simulink model "three_phase_full_wave_fully_controlled_rectifier_ckt_for_seperately_exiceted_dc_motor"  (R2025a)
settings: Solver=VariableStepAuto  StartTime=0.0  StopTime=.1  RelTol=1e-3
libraries: spsThyristorLib x6, spsDCVoltageSourceLib x1, spsCurrentMeasurementLib x1, spsSeriesRLCBranchLib x1, spsThreePhaseVIMeasurementLib x1, spsThreePhaseSourceLib x1, spsVoltageMeasurementLib x1, sps_lib x1
settings Model: Creator=HP  LastModifiedBy=samar

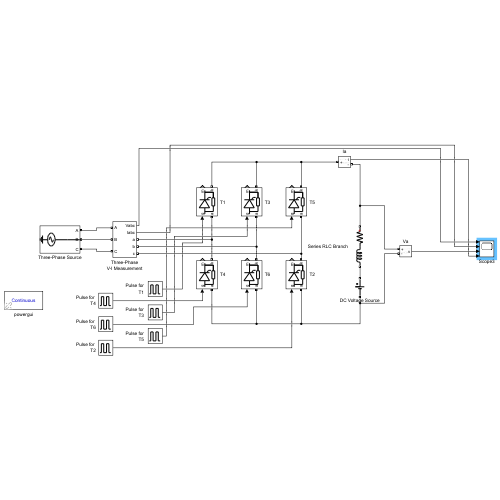
[thumbnail: Simulink's stored preview of the top-level diagram]
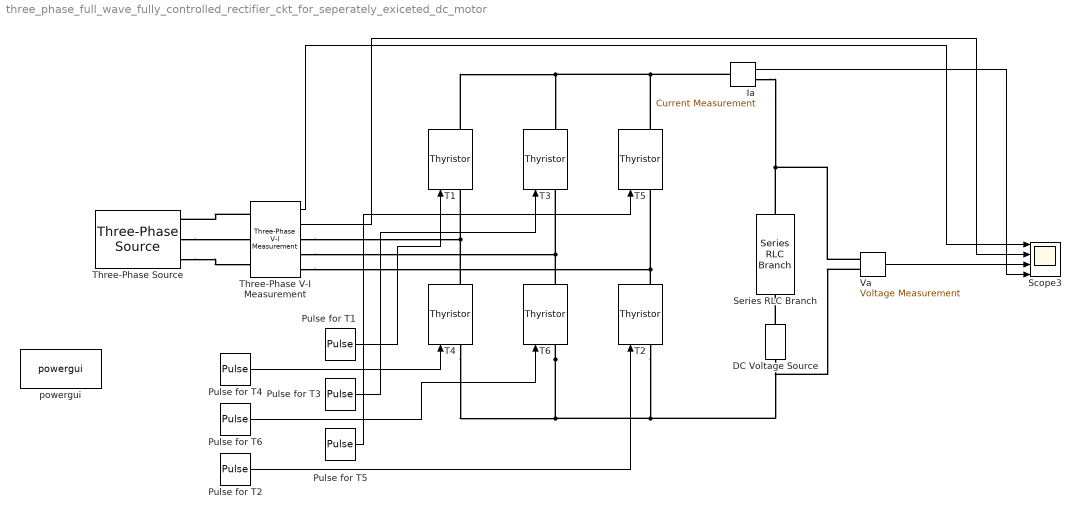
== system three_phase_full_wave_fully_controlled_rectifier_ckt_for_seperately_exiceted_dc_motor ==
  DC Voltage Source : spsDCVoltageSourceLib/DC Voltage Source  Amplitude=100  Measurements=None
  Ia : spsCurrentMeasurementLib/Current Measurement  PhasorSimulation=off  OutputType=Complex  PSBequivalent=0
  "Pulse for T1 " : DiscretePulseGenerator  PulseType=Time based  Amplitude=5  Period=1/50  PulseWidth=120/360*100  PhaseDelay=(30/360)*0.02
  Pulse for T2 : DiscretePulseGenerator  PulseType=Time based  Amplitude=5  Period=1/50  PulseWidth=33.33333333  PhaseDelay=(90/360)*0.02
  "Pulse for T3 " : DiscretePulseGenerator  PulseType=Time based  Amplitude=5  Period=1/50  PulseWidth=33.33333333  PhaseDelay=(150/360)*0.02
  Pulse for T4 : DiscretePulseGenerator  PulseType=Time based  Amplitude=5  Period=1/50  PulseWidth=33.33333333  PhaseDelay=(210/360)*0.02
  "Pulse for T5 " : DiscretePulseGenerator  PulseType=Time based  Amplitude=5  Period=1/50  PulseWidth=33.33333333  PhaseDelay=(270/360)*0.02
  Pulse for T6 : DiscretePulseGenerator  PulseType=Time based  Amplitude=5  Period=1/50  PulseWidth=33.3333333  PhaseDelay=(330/360)*0.02
  Scope3 : Scope  NumInputPorts=4
      settings: ActiveDisplayYMinimum=-423.55759863102935  ActiveDisplayYMaximum=423.55760105345479  DataLoggingVariableName=ScopeData3
  Series RLC Branch : spsSeriesRLCBranchLib/Series RLC Branch  LConnTagsString=__new0  RConnTagsString=__new0  BranchType=RL  Resistance=1  Inductance=10e-3  SetiL0=off  InitialCurrent=0  Capacitance=1e-6  Setx0=off  InitialVoltage=0  Measurements=None
  T{1..6} (6 alike) : spsThyristorLib/Thyristor  Ron=0.001  Lon=0  Vf=0.8  IC=0  Rs=500  Cs=250e-9  Measurements=on
  Three-Phase V-I Measurement : spsThreePhaseVIMeasurementLib/Three-Phase V-I Measurement  VoltageMeasurement=phase-to-ground  SetLabelV=off  LabelV=Vabc  Vpu=off  VpuLL=off  CurrentMeasurement=yes  SetLabelI=off  LabelI=Iabc  Ipu=off  Pbase=100e6  Vbase=500e3  OutputType=Complex  PhasorSimulation=off  PSBequivalent=0
  Three-Phase Source : spsThreePhaseSourceLib/Three-Phase Source  InternalConnection=Yg  VoltagePhases=off  Voltage=415  PhaseAngle=0  Voltage_phases=[25e3 25e3 25e3]/sqrt(3)  PhaseAngles_phases=[0 -120 +120]  Frequency=50  NonIdealSource=off  SpecifyImpedance=off  Resistance=0.8929  Inductance=16.58e-3  ShortCircuitLevel=100e6  BaseVoltage=25e3  XRratio=7  BusType=swing  Pref=10e3  Qref=0  Prefabc=[10e3, 10e3, 10e3]  Qrefabc=[0, 0, 0]  Qmin=-inf  Qmax=inf
  Va : spsVoltageMeasurementLib/Voltage Measurement  PhasorSimulation=off  OutputType=Complex  PSBequivalent=0
  powergui : sps_lib/powergui  Priority=1  SimulationMode=Continuous  SampleTime=50e-6  frequency=60  Iterations=50  frequencyindice=50  Pbase=100e6  ErrMax=1e-4  UnitsV=kV  UnitsW=MW  buscounter=0  FunctionMessages=off  echomessages=off  EnableUseOfTLC=off  CurrentSourceSwitches=off  DisableSnubberDevices=off  DisableRonSwitches=off  DisableVfSwitches=off  DisplayEquations=off  AutomaticDiscreteSolvers=off  SolverType=Tustin/Backward Euler (TBE)  Interpol=off  ExternalGateDelay=off  methode=off  Ts=100  x0status=blocks  SPID=on  SwTol=0  HookPort=off  NonlinearTolerance=1e-4  nMaxIteration=100  ContinueOnMaxIteration=off  RestoreLinks=warning  ResistiveCurrentMeasurement=off  Frange=[0:2:500]  Ylog=off  Xlog=on  ShowGrid=off  save=off  variable=ZData  structure=0  ZoomFFT=off  StartTime=0.0  cycles=1  DisplayStyle=1  fundamental=60  FreqAxis=off  MaxFrequency=1000  frequencyindicesteady=1  RmsSteady=1  display=off
  wires:
  "Pulse for T3 "/1 -> T3/1
  "Pulse for T1 "/1 -> T1/1
  Ia/1 -> Scope3/4
  Va/1 -> Scope3/3
  "Pulse for T5 "/1 -> T5/1
  Three-Phase V-I Measurement/1 -> Scope3/1
  Three-Phase V-I Measurement/2 -> Scope3/2
  Pulse for T4/1 -> T4/1
  Pulse for T2/1 -> T2/1
  Pulse for T6/1 -> T6/1
  connections:
  T4/RConn1 -- T1/LConn1 -- Three-Phase V-I Measurement/RConn1
  Ia/LConn1 -- T5/RConn1 -- T1/RConn1 -- T3/RConn1
  T6/RConn1 -- Three-Phase V-I Measurement/RConn2 -- T3/LConn1
  T6/LConn1 -- DC Voltage Source/LConn1 -- Va/LConn2 -- T2/LConn1 -- T4/LConn1
  Ia/RConn1 -- Va/LConn1 -- Series RLC Branch/LConn1
  DC Voltage Source/RConn1 -- Series RLC Branch/RConn1
  T2/RConn1 -- T5/LConn1 -- Three-Phase V-I Measurement/RConn3
  Three-Phase V-I Measurement/LConn1 -- Three-Phase Source/RConn1
  Three-Phase Source/RConn2 -- Three-Phase V-I Measurement/LConn2
  Three-Phase Source/RConn3 -- Three-Phase V-I Measurement/LConn3
